simulink model "partage_RSV"  (Simulink 7.5)
settings: Solver=ode45  StartTime=0.0  StopTime=10.0  RelTol=1e-3
settings Model: Creator=paris  LastModifiedBy=paris

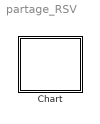
== system partage_RSV ==
  Chart : Stateflow chart  TreatAsAtomicUnit=on

== stateflow chart Chart ==
  state Risque_Sortie_Voie
    state Dans_Voie
    state SV_Possible
    state SV_Imminente
    state SV_Effective
    (default) -> Dans_Voie
    SV_Effective -> Dans_Voie : [ml.etat_SV==0]
    Dans_Voie -> SV_Possible : [ml.tlcCalcule<=3]
    SV_Possible -> SV_Imminente : [ml.tlcCalcule<=1.5]
    SV_Imminente -> SV_Effective : [ml.tlcCalcule<=0]
